simulink model "Pacemaker_final"  (R2020a)
settings: Solver=FixedStepAuto  StartTime=0.0  StopTime=10.0  FixedStep=1e-3  RelTol=1e-3  EnableMultiTasking=on
libraries: etargetslib x17, frdmk64flib x7, simulink x1
(part 1 of 3)
settings Model: ExtModeTrigDuration=5  Creator=Tim_G  LastModifiedBy=Tim_G
settings OptimizationCC: EnhancedBackFolding=on  PassReuseOutputArgsAs=Individual arguments  ZeroExternalMemoryAtStartup=off  ZeroInternalMemoryAtStartup=off  MaxStackSize=64  OptimizeBlockOrder=speed  DifferentSizesBufferReuse=on  OptimizationCustomize=off  EfficientTunableParamExpr=on
settings DebuggingCC: ParameterTunabilityLossMsg=error
settings HardwareCC: ProdBitPerPointer=32  ProdBitPerSizeT=32  ProdBitPerPtrDiffT=32  ProdLargestAtomicInteger=Long  ProdLargestAtomicFloat=Double  ProdEndianess=BigEndian  ProdWordSize=32  ProdHWDeviceType=ARM Compatible->ARM Cortex
settings SFSimCC: MATLABDynamicMemAlloc=off
settings RTWCC: SystemTargetFile=ert.tlc  HardwareBoard=NXP FRDM-K64F  TemplateMakefile=ert_default_tmf  Toolchain=GNU Tools for ARM Embedded Processors
settings CodeAppCC: ForceParamTrailComments=on  IgnoreCustomStorageClasses=off  OperatorAnnotations=on  SimulinkDataObjDesc=on  SFDataObjDesc=on  InsertBlockDesc=on

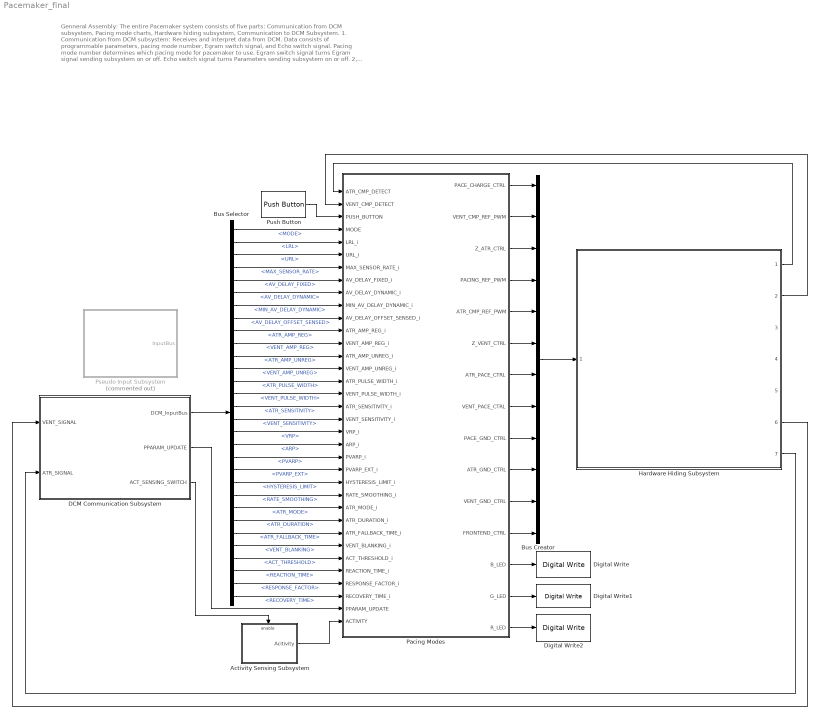
== system Pacemaker_final ==
  note: Genneral Assembly:
      |  The entire Pacemaker system consists of five parts: Communication from DCM subsystem, Pacing mode charts, Hardware hiding subsystem, Communication to DCM Subsystem.
      | 1. Communication from DCM subsystem:
      |       Receives and interpret data from DCM. Data consists of programmable parameters, pacing mode number, Egram switch signal, and Echo switch signal.
      |       Pacing mode number determines which pacing mode for pacemaker to use.
      |       Egram switch signal turns Egram signal sending subsystem on or off.
      |       Echo switch signal turns Parameters sending subsystem on or off.
      | 2, Pacing Modes subsystem:
      |       Implementation of different pacing methods. A multiport switch chooses from which pacing mode to output control signals.
      | 3. Hardware hiding subsystem:
      |       Takes control signals as inputs and sends them to the hardware. Also outputs signals received from the hardware.
      | 4. Communication to DCM Subsystem:
      | 	Sends programmable parameters and/or egram signals to DCM if enable signals (ECHO and/or EGRAM) are turned on.
  Activity Sensing Subsystem : Subsystem
  Bus Creator : BusCreator  Inputs=12
  Bus Selector : BusSelector  OutputSignals=MODE,LRL,URL,MAX_SENSOR_RATE,AV_DELAY_FIXED,AV_DELAY_DYNAMIC,MIN_AV_DELAY_DYNAMIC,AV_DELAY_OFFSET_SENSED,ATR_AMP_REG,VENT_AMP_REG,ATR_AMP_UNREG,VENT_AMP_UNREG,ATR_PULSE_WIDTH,VENT_PULSE_WIDTH,ATR_SENSITIVITY,VENT_SENSITIVITY,VRP,ARP,PVARP,PVARP_EXT,HYSTERESIS_LIMIT,RATE_SMOOTHING,ATR_MODE,ATR_DURATION,ATR_FALLBACK_TIME,VENT_BLANKING,ACT_THRESHOLD,REACTION_TIME,RESPONSE_FACTOR,RECOVERY_TIME
  DCM Communication Subsystem : Subsystem
  Digital Write : frdmk64flib/Digital Write  Whichpin=BLUE_LED
  Digital Write1 : frdmk64flib/Digital Write  Whichpin=GREEN_LED
  Digital Write2 : frdmk64flib/Digital Write  Whichpin=RED_LED
  Hardware Hiding Subsystem : Subsystem  ReferencedSubsystem=k64f_hardware_subsystem
  Pacing Modes : Stateflow chart  TreatAsAtomicUnit=on
      settings: PortSchema="{\"entries\":[{\"content\":{\"sides\":[{\"content\":{\"connectorIds\":[\"In2\",\"In1\",\"In3\",\"In4\",\"In5\",\"In6\",\"In7\",\"In8\",\"In9\",\"In10\",\"In11\",\"In12\",\"In13\",\"In14\",\"In15\",\"In16\",\"In17\",\"In18\",\"In19\",\"In20\",\"In21\",\"In22\",\"In23\",\"In24\",\"In25\",\"In26\",\"In27\",\"In28\",\"In29\",\"In30\",\"In31\",\"In32\",\"In33\",\"In34\",\"In35\"]},\"type\":\"ConnectorPlacement.EquallySpacedRectSide\",\"uuid\":\"6566e723-a8a5-46a2-b90e-16d152fbfa35\"},{\"content\":{\"connectorIds\":[\"Out1\",\"Out2\",\"Out3\",\"Out4\",\"Out5\",\"Out6\",\"Out7\",\"Out8\",\"Out9\",\"Out10\",\"Out11\",\"Out12\",\"Out13\",\"Out14\",\"Out15\"],\"side\":\"RIGHT\"},\"type\":\"ConnectorPlacement.EquallySpacedRectSide\",\"uuid\":\"5fe4a0a7-04e7-4415-b3ec-d211b0e34153\"},{\"content\":{\"connectorIds\":[],\"side\":\"TOP\"},\"type\":\"ConnectorPlacement.EquallySpacedRectSide\",\"uuid\":\"941869fe-4fac-4529-93d8-39aa0ba9c0c9\"}]},\"type\":\"ConnectorPlacement.EquallySpacedConnector\",\"uuid\":\"3c081651-2393-41e1-9361-10a041cf70c8\"}],\"packageUris\":[\"http://schema.mathworks.com/mf0/Connector/19700101\"],\"version\":\"1.0\"}"
  Pseudo Input Subsystem : Subsystem  Commented=on
  Push Button : frdmk64flib/Push Button  Whichswitch=SW2  SampleTime1=-1
  wires:
  Hardware Hiding Subsystem/7 -> DCM Communication Subsystem/2(ATR_SIGNAL)
  Hardware Hiding Subsystem/6 -> DCM Communication Subsystem/1(VENT_SIGNAL)
  Push Button/1 -> Pacing Modes/3(PUSH_BUTTON)
  Hardware Hiding Subsystem/2 -> Pacing Modes/1(VENT_CMP_DETECT)
  Hardware Hiding Subsystem/1 -> Pacing Modes/2(ATR_CMP_DETECT)
  Pacing Modes/1(PACE_CHARGE_CTRL) -> Bus Creator/1
  Pacing Modes/2(VENT_CMP_REF_PWM) -> Bus Creator/2
  Pacing Modes/3(Z_ATR_CTRL) -> Bus Creator/3
  Pacing Modes/4(PACING_REF_PWM) -> Bus Creator/4
  Pacing Modes/5(ATR_CMP_REF_PWM) -> Bus Creator/5
  Pacing Modes/6(Z_VENT_CTRL) -> Bus Creator/6
  Pacing Modes/7(ATR_PACE_CTRL) -> Bus Creator/7
  Pacing Modes/8(VENT_PACE_CTRL) -> Bus Creator/8
  Pacing Modes/9(PACE_GND_CTRL) -> Bus Creator/9
  Pacing Modes/10(ATR_GND_CTRL) -> Bus Creator/10
  Pacing Modes/11(VENT_GND_CTRL) -> Bus Creator/11
  Pacing Modes/12(FRONTEND_CTRL) -> Bus Creator/12
  Bus Creator/1 -> Hardware Hiding Subsystem/1
  DCM Communication Subsystem/1(DCM_InputBus) -> Bus Selector/1
  Bus Selector/1 -> Pacing Modes/4(MODE)  "<MODE>"
  Bus Selector/2 -> Pacing Modes/5(LRL_i)  "<LRL>"
  Bus Selector/3 -> Pacing Modes/6(URL_i)  "<URL>"
  Bus Selector/4 -> Pacing Modes/7(MAX_SENSOR_RATE_i)  "<MAX_SENSOR_RATE>"
  Bus Selector/5 -> Pacing Modes/8(AV_DELAY_FIXED_i)  "<AV_DELAY_FIXED>"
  Bus Selector/6 -> Pacing Modes/9(AV_DELAY_DYNAMIC_i)  "<AV_DELAY_DYNAMIC>"
  Bus Selector/7 -> Pacing Modes/10(MIN_AV_DELAY_DYNAMIC_i)  "<MIN_AV_DELAY_DYNAMIC>"
  Bus Selector/8 -> Pacing Modes/11(AV_DELAY_OFFSET_SENSED_i)  "<AV_DELAY_OFFSET_SENSED>"
  Bus Selector/9 -> Pacing Modes/12(ATR_AMP_REG_i)  "<ATR_AMP_REG>"
  Bus Selector/10 -> Pacing Modes/13(VENT_AMP_REG_i)  "<VENT_AMP_REG>"
  Bus Selector/11 -> Pacing Modes/14(ATR_AMP_UNREG_i)  "<ATR_AMP_UNREG>"
  Bus Selector/12 -> Pacing Modes/15(VENT_AMP_UNREG_i)  "<VENT_AMP_UNREG>"
  Bus Selector/13 -> Pacing Modes/16(ATR_PULSE_WIDTH_i)  "<ATR_PULSE_WIDTH>"
  Bus Selector/14 -> Pacing Modes/17(VENT_PULSE_WIDTH_i)  "<VENT_PULSE_WIDTH>"
  Bus Selector/15 -> Pacing Modes/18(ATR_SENSITIVITY_i)  "<ATR_SENSITIVITY>"
  Bus Selector/16 -> Pacing Modes/19(VENT_SENSITIVITY_i)  "<VENT_SENSITIVITY>"
  Bus Selector/17 -> Pacing Modes/20(VRP_i)  "<VRP>"
  Bus Selector/18 -> Pacing Modes/21(ARP_i)  "<ARP>"
  Bus Selector/19 -> Pacing Modes/22(PVARP_i)  "<PVARP>"
  Bus Selector/20 -> Pacing Modes/23(PVARP_EXT_i)  "<PVARP_EXT>"
  Bus Selector/21 -> Pacing Modes/24(HYSTERESIS_LIMIT_i)  "<HYSTERESIS_LIMIT>"
  Bus Selector/22 -> Pacing Modes/25(RATE_SMOOTHING_i)  "<RATE_SMOOTHING>"
  Bus Selector/23 -> Pacing Modes/26(ATR_MODE_i)  "<ATR_MODE>"
  Bus Selector/24 -> Pacing Modes/27(ATR_DURATION_i)  "<ATR_DURATION>"
  Bus Selector/25 -> Pacing Modes/28(ATR_FALLBACK_TIME_i)  "<ATR_FALLBACK_TIME>"
  Bus Selector/26 -> Pacing Modes/29(VENT_BLANKING_i)  "<VENT_BLANKING>"
  Bus Selector/27 -> Pacing Modes/30(ACT_THRESHOLD_i)  "<ACT_THRESHOLD>"
  Bus Selector/28 -> Pacing Modes/31(REACTION_TIME_i)  "<REACTION_TIME>"
  Bus Selector/29 -> Pacing Modes/32(RESPONSE_FACTOR_i)  "<RESPONSE_FACTOR>"
  Bus Selector/30 -> Pacing Modes/33(RECOVERY_TIME_i)  "<RECOVERY_TIME>"
  Pacing Modes/13(B_LED) -> Digital Write/1
  Pacing Modes/14(G_LED) -> Digital Write1/1
  Pacing Modes/15(R_LED) -> Digital Write2/1
  DCM Communication Subsystem/2(PPARAM_UPDATE) -> Pacing Modes/34(PPARAM_UPDATE)
  Activity Sensing Subsystem/1(Acitivity) -> Pacing Modes/35(ACTIVITY)
  DCM Communication Subsystem/3(ACT_SENSING_SWITCH) -> Activity Sensing Subsystem/Enable

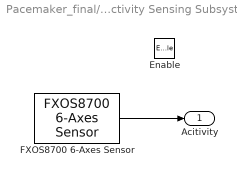
== system Pacemaker_final/Activity Sensing Subsystem ==
  Enable : EnablePort
  FXOS8700 6-Axes Sensor : frdmk64flib/FXOS8700 6-Axes Sensor  Activesensor=Accelerometer only  ODR=800Hz  HybridODR=400Hz  Accelfullrange=-2g to +2g  SampleTime=0.01
  Acitivity : Outport
  wires:
  FXOS8700 6-Axes Sensor/1 -> Acitivity/1

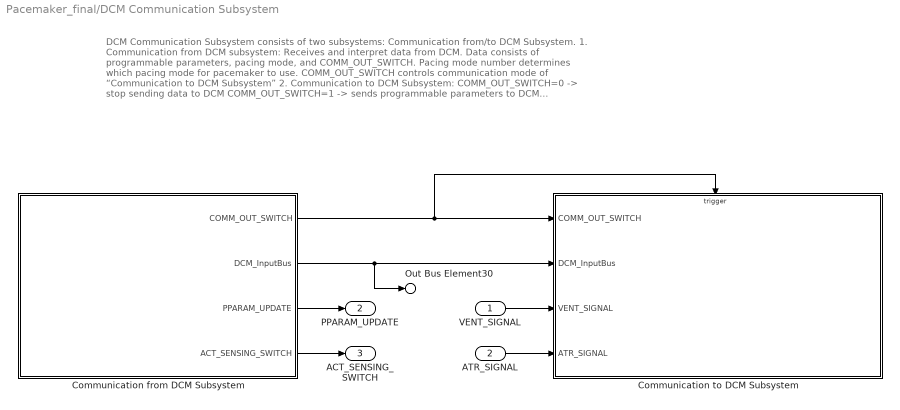
== system Pacemaker_final/DCM Communication Subsystem ==
  note: DCM Communication Subsystem consists of two subsystems: Communication from/to DCM Subsystem.
      | 1. Communication from DCM subsystem:
      | Receives and interpret data from DCM.
      | Data consists of programmable parameters, pacing mode, and COMM_OUT_SWITCH.
      | Pacing mode number determines which pacing mode for pacemaker to use.
      | COMM_OUT_SWITCH controls communication mode of “Communication to DCM Subsystem”
      | 2. Communication to DCM Subsystem:
      | COMM_OUT_SWITCH=0 -> stop sending data to DCM
      | COMM_OUT_SWITCH=1 -> sends programmable parameters to DCM
      | COMM_OUT_SWITCH=2 -> s ends egram signals to DCM
  VENT_SIGNAL : Inport  OutDataTypeStr=double
  ATR_SIGNAL : Inport  Port=2  OutDataTypeStr=double
  Communication from DCM Subsystem : Subsystem
  Communication to DCM Subsystem : Subsystem  TreatAsAtomicUnit=on
  Out Bus Element30 : Outport  PortName=DCM_InputBus
  PPARAM_UPDATE : Outport  Port=2
  ACT_SENSING_SWITCH : Outport  Port=3
  wires:
  VENT_SIGNAL/1 -> Communication to DCM Subsystem/3(VENT_SIGNAL)
  ATR_SIGNAL/1 -> Communication to DCM Subsystem/4(ATR_SIGNAL)
  Communication from DCM Subsystem/3(PPARAM_UPDATE) -> PPARAM_UPDATE/1
  Communication from DCM Subsystem/1(COMM_OUT_SWITCH) -> Communication to DCM Subsystem/Trigger, Communication to DCM Subsystem/1(COMM_OUT_SWITCH)
  Communication from DCM Subsystem/4(ACT_SENSING_SWITCH) -> ACT_SENSING_SWITCH/1
  Communication from DCM Subsystem/2(DCM_InputBus) -> Out Bus Element30/1, Communication to DCM Subsystem/2(DCM_InputBus)

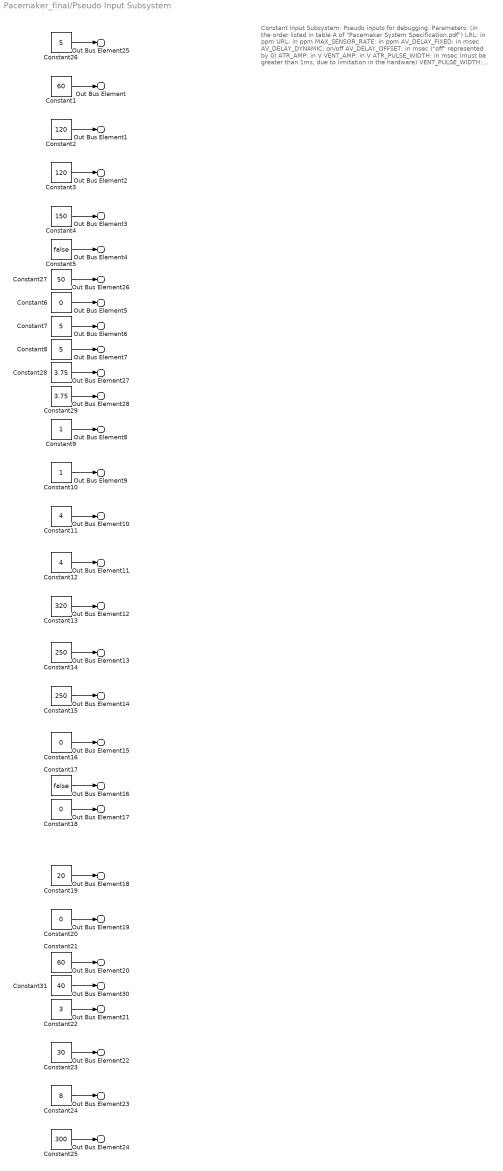
== system Pacemaker_final/Pseudo Input Subsystem ==
  note: Constant Input Subsystem:
      | Pseudo inputs for debugging.
      |
      | Parameters:
      | (in the order listed in table A of "Pacemaker System Specification.pdf")
      | LRL: in ppm
      | URL: in ppm
      | MAX_SENSOR_RATE: in ppm
      | AV_DELAY_FIXED: in msec
      | AV_DELAY_DYNAMIC: on/off
      | AV_DELAY_OFFSET: in msec ("off" represented by 0)
      | ATR_AMP: in V
      | VENT_AMP: in V
      | ATR_PULSE_WIDTH: in msec (must be greater than 1ms, due to
      | limitation in the hardware)
      | VENT_PULSE_WIDTH: in msec
      | ATR_SENSITIVITY: in V
      | VENT_SENSITIVITY: in V
      | VRP: in msec
      | ARP: in msec
      | PVARP: in msec
      | PVARP_EXT: in msec ("off" represented by 0)
      | HYSTERESIS: off/same choices as LRL (represented by "on")
      | RATE_SMOOTHING: off represented by 0
      | ATR_DURATION: in cardiac cycles
      | ATR_FALLBACK_MODE
      | ATR_FALLBACK_TIME: in sec
      | ACT_THRESHOLD:
      | 0-V-Low
      | 1-Low
      | 2-Med-Low
      | 3-Med
      | 4-Med-High
      | 5-High
      | 6-V-High
      | REACTION_TIME: in sec
      | RESPONSE_FACTOR
      | RECOVERY_TIME: in sec
  Constant1 : Constant  Value=60
  Constant10 : Constant
  Constant11 : Constant  Value=4
  Constant12 : Constant  Value=4
  Constant13 : Constant  Value=320
  Constant14 : Constant  Value=250
  Constant15 : Constant  Value=250
  Constant{6,16,18,20} (4 alike) : Constant  Value=0
  Constant17 : Constant  Value=false
  Constant19 : Constant  Value=20
  Constant2 : Constant  Value=120
  Constant21 : Constant  Value=60
  Constant22 : Constant  Value=3
  Constant23 : Constant  Value=30
  Constant24 : Constant  Value=8
  Constant25 : Constant  Value=300
  Constant26 : Constant  Value=5
  Constant27 : Constant  Value=50
  Constant28 : Constant  Value=3.75
  Constant29 : Constant  Value=3.75
  Constant3 : Constant  Value=120
  Constant31 : Constant  Value=40
  Constant4 : Constant  Value=150
  Constant5 : Constant  Value=false
  Constant7 : Constant  Value=5
  Constant8 : Constant  Value=5
  Constant9 : Constant
  Out Bus Element : Outport  PortName=InputBus  Element=LRL
  Out Bus Element1 : Outport  PortName=InputBus  Element=URL
  Out Bus Element2 : Outport  PortName=InputBus  Element=MAX_SENSOR_RATE
  Out Bus Element3 : Outport  PortName=InputBus  Element=AV_DELAY_FIXED
  Out Bus Element4 : Outport  PortName=InputBus  Element=AV_DELAY_DYNAMIC
  Out Bus Element5 : Outport  PortName=InputBus  Element=AV_DELAY_OFFSET_SENSED
  Out Bus Element6 : Outport  PortName=InputBus  Element=ATR_AMP_REG
  Out Bus Element7 : Outport  PortName=InputBus  Element=VENT_AMP_REG
  Out Bus Element8 : Outport  PortName=InputBus  Element=ATR_PULSE_WIDTH
  Out Bus Element9 : Outport  PortName=InputBus  Element=VENT_PULSE_WIDTH
  Out Bus Element10 : Outport  PortName=InputBus  Element=ATR_SENSITIVITY
  Out Bus Element11 : Outport  PortName=InputBus  Element=VENT_SENSITIVITY
  Out Bus Element12 : Outport  PortName=InputBus  Element=VRP
  Out Bus Element13 : Outport  PortName=InputBus  Element=ARP
  Out Bus Element14 : Outport  PortName=InputBus  Element=PVARP
  Out Bus Element15 : Outport  PortName=InputBus  Element=PVARP_EXT
  Out Bus Element16 : Outport  PortName=InputBus  Element=HYSTERESIS
  Out Bus Element17 : Outport  PortName=InputBus  Element=RATE_SMOOTHING
  Out Bus Element18 : Outport  PortName=InputBus  Element=ATR_DURATION
  Out Bus Element19 : Outport  PortName=InputBus  Element=ATR_FALLBACK_MODE
  Out Bus Element20 : Outport  PortName=InputBus  Element=ATR_FALLBACK_TIME
  Out Bus Element21 : Outport  PortName=InputBus  Element=ACT_THRESHOLD
  Out Bus Element22 : Outport  PortName=InputBus  Element=REACTION_TIME
  Out Bus Element23 : Outport  PortName=InputBus  Element=RESPONSE_FACTOR
  Out Bus Element24 : Outport  PortName=InputBus  Element=RECOVERY_TIME
  Out Bus Element25 : Outport  PortName=InputBus  Element=MODE
  Out Bus Element26 : Outport  PortName=InputBus  Element=MIN_AV_DELAY_DYNAMIC
  Out Bus Element27 : Outport  PortName=InputBus  Element=ATR_AMP_UNREG
  Out Bus Element28 : Outport  PortName=InputBus  Element=VENT_AMP_UNREG
  Out Bus Element30 : Outport  PortName=InputBus  Element=VENT_BLANKING
  wires:
  Constant1/1 -> Out Bus Element/1
  Constant2/1 -> Out Bus Element1/1
  Constant4/1 -> Out Bus Element3/1
  Constant3/1 -> Out Bus Element2/1
  Constant5/1 -> Out Bus Element4/1
  Constant6/1 -> Out Bus Element5/1
  Constant8/1 -> Out Bus Element7/1
  Constant7/1 -> Out Bus Element6/1
  Constant10/1 -> Out Bus Element9/1
  Constant11/1 -> Out Bus Element10/1
  Constant9/1 -> Out Bus Element8/1
  Constant13/1 -> Out Bus Element12/1
  Constant12/1 -> Out Bus Element11/1
  Constant14/1 -> Out Bus Element13/1
  Constant15/1 -> Out Bus Element14/1
  Constant19/1 -> Out Bus Element18/1
  Constant18/1 -> Out Bus Element17/1
  Constant16/1 -> Out Bus Element15/1
  Constant17/1 -> Out Bus Element16/1
  Constant25/1 -> Out Bus Element24/1
  Constant24/1 -> Out Bus Element23/1
  Constant23/1 -> Out Bus Element22/1
  Constant22/1 -> Out Bus Element21/1
  Constant20/1 -> Out Bus Element19/1
  Constant21/1 -> Out Bus Element20/1
  Constant26/1 -> Out Bus Element25/1
  Constant27/1 -> Out Bus Element26/1
  Constant28/1 -> Out Bus Element27/1
  Constant29/1 -> Out Bus Element28/1
  Constant31/1 -> Out Bus Element30/1

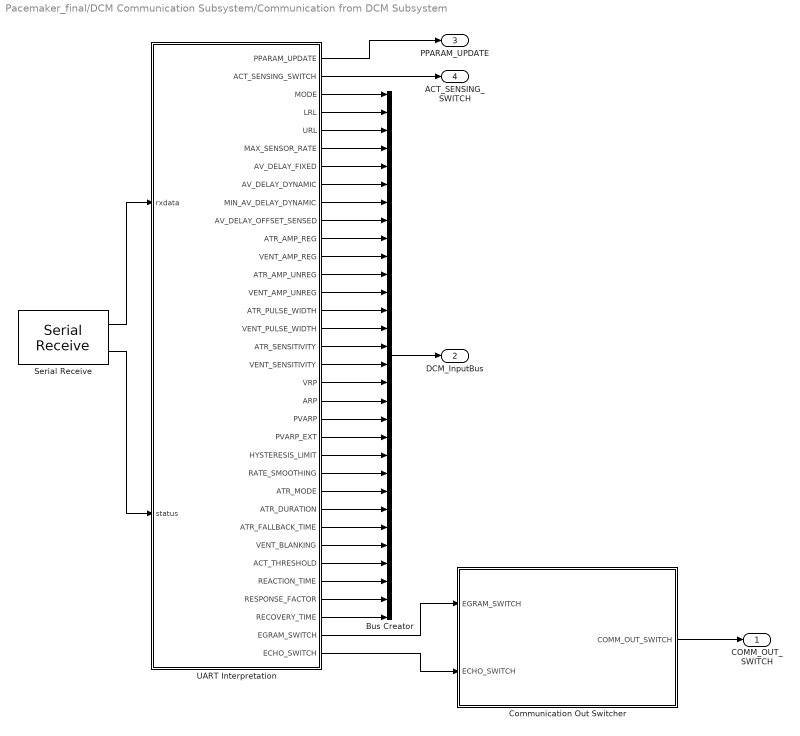
== system Pacemaker_final/DCM Communication Subsystem/Communication from DCM Subsystem ==
  Bus Creator : BusCreator  Inputs=30
  Communication Out Switcher : Stateflow chart  TreatAsAtomicUnit=on
  Serial Receive : frdmk64flib/Serial Receive  SCIModule=0  Baudrate=uint32(9600)  Parity=None  StopBits=1  HardwareFlowControl=None  ByteOrder=LittleEndian  DataType=uint8  DataLength=59  BlockingMode=off  OutputStatus=on  SampleTime=-1
  UART Interpretation : Stateflow chart  TreatAsAtomicUnit=on
      settings: PortSchema="{\"entries\":[{\"content\":{\"sides\":[{\"content\":{\"connectorIds\":[\"In1\",\"In2\"]},\"type\":\"ConnectorPlacement.EquallySpacedRectSide\",\"uuid\":\"8bf45b7e-957d-4d49-8afa-52d597e5211b\"},{\"content\":{\"connectorIds\":[\"Out33\",\"Out34\",\"Out1\",\"Out2\",\"Out3\",\"Out4\",\"Out5\",\"Out6\",\"Out7\",\"Out8\",\"Out9\",\"Out10\",\"Out11\",\"Out12\",\"Out13\",\"Out14\",\"Out15\",\"Out16\",\"Out17\",\"Out18\",\"Out19\",\"Out20\",\"Out21\",\"Out22\",\"Out23\",\"Out24\",\"Out25\",\"Out26\",\"Out27\",\"Out28\",\"Out29\",\"Out30\",\"Out31\",\"Out32\"],\"side\":\"RIGHT\"},\"type\":\"ConnectorPlacement.EquallySpacedRectSide\",\"uuid\":\"d38d0b56-01b9-48e9-aa1c-1551120d845a\"},{\"content\":{\"connectorIds\":[],\"side\":\"TOP\"},\"type\":\"ConnectorPlacement.EquallySpacedRectSide\",\"uuid\":\"18196cd6-21fd-4409-aed1-274194e36cea\"}]},\"type\":\"ConnectorPlacement.EquallySpacedConnector\",\"uuid\":\"d120a801-f3dc-4c99-bead-ec7f8e612754\"}],\"packageUris\":[\"http://schema.mathworks.com/mf0/Connector/19700101\"],\"version\":\"1.0\"}"
  COMM_OUT_SWITCH : Outport
  DCM_InputBus : Outport  Port=2
  PPARAM_UPDATE : Outport  Port=3
  ACT_SENSING_SWITCH : Outport  Port=4
  wires:
  UART Interpretation/5(AV_DELAY_FIXED) -> Bus Creator/5
  UART Interpretation/14(VENT_PULSE_WIDTH) -> Bus Creator/14
  UART Interpretation/10(VENT_AMP_REG) -> Bus Creator/10
  UART Interpretation/17(VRP) -> Bus Creator/17
  UART Interpretation/6(AV_DELAY_DYNAMIC) -> Bus Creator/6
  UART Interpretation/9(ATR_AMP_REG) -> Bus Creator/9
  UART Interpretation/27(ACT_THRESHOLD) -> Bus Creator/27
  UART Interpretation/24(ATR_DURATION) -> Bus Creator/24
  UART Interpretation/18(ARP) -> Bus Creator/18
  UART Interpretation/8(AV_DELAY_OFFSET_SENSED) -> Bus Creator/8
  UART Interpretation/7(MIN_AV_DELAY_DYNAMIC) -> Bus Creator/7
  Serial Receive/2 -> UART Interpretation/2(status)
  UART Interpretation/3(URL) -> Bus Creator/3
  UART Interpretation/26(VENT_BLANKING) -> Bus Creator/26
  UART Interpretation/13(ATR_PULSE_WIDTH) -> Bus Creator/13
  UART Interpretation/15(ATR_SENSITIVITY) -> Bus Creator/15
  UART Interpretation/11(ATR_AMP_UNREG) -> Bus Creator/11
  UART Interpretation/16(VENT_SENSITIVITY) -> Bus Creator/16
  UART Interpretation/30(RECOVERY_TIME) -> Bus Creator/30
  UART Interpretation/20(PVARP_EXT) -> Bus Creator/20
  UART Interpretation/29(RESPONSE_FACTOR) -> Bus Creator/29
  UART Interpretation/19(PVARP) -> Bus Creator/19
  Serial Receive/1 -> UART Interpretation/1(rxdata)
  UART Interpretation/4(MAX_SENSOR_RATE) -> Bus Creator/4
  UART Interpretation/23(ATR_MODE) -> Bus Creator/23
  UART Interpretation/22(RATE_SMOOTHING) -> Bus Creator/22
  UART Interpretation/12(VENT_AMP_UNREG) -> Bus Creator/12
  UART Interpretation/28(REACTION_TIME) -> Bus Creator/28
  UART Interpretation/25(ATR_FALLBACK_TIME) -> Bus Creator/25
  UART Interpretation/21(HYSTERESIS_LIMIT) -> Bus Creator/21
  UART Interpretation/2(LRL) -> Bus Creator/2
  UART Interpretation/1(MODE) -> Bus Creator/1
  Bus Creator/1 -> DCM_InputBus/1
  Communication Out Switcher/1(COMM_OUT_SWITCH) -> COMM_OUT_SWITCH/1
  UART Interpretation/31(EGRAM_SWITCH) -> Communication Out Switcher/1(EGRAM_SWITCH)
  UART Interpretation/32(ECHO_SWITCH) -> Communication Out Switcher/2(ECHO_SWITCH)
  UART Interpretation/33(PPARAM_UPDATE) -> PPARAM_UPDATE/1
  UART Interpretation/34(ACT_SENSING_SWITCH) -> ACT_SENSING_SWITCH/1

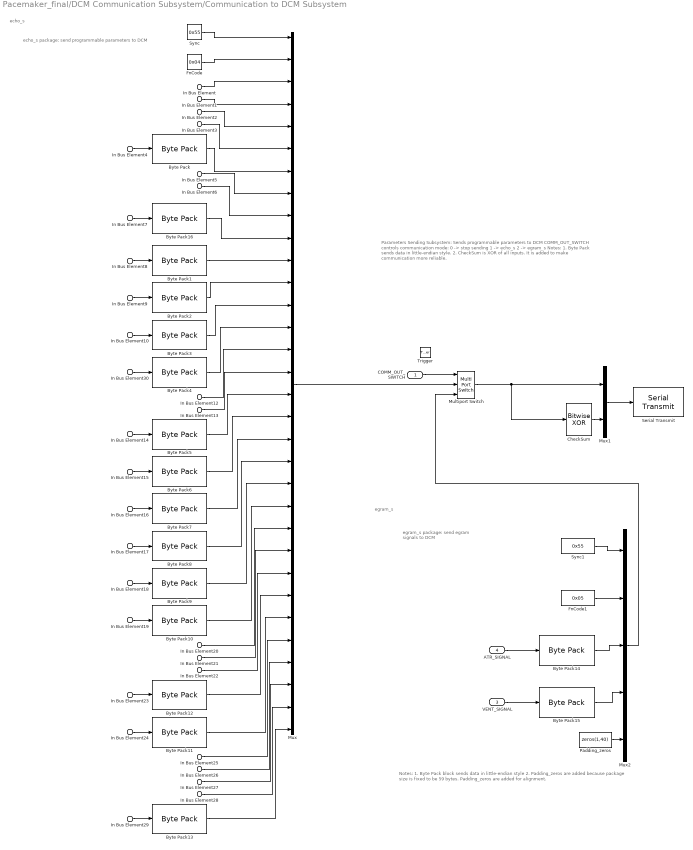
== system Pacemaker_final/DCM Communication Subsystem/Communication to DCM Subsystem ==
  note: egram_s package:
      | send egram signals to DCM
  note: echo_s package:
      | send programmable parameters to DCM
  note: echo_s
  note: egram_s
  note: Parameters Sending Subsystem:
      | Sends programmable parameters to DCM
      | COMM_OUT_SWITCH controls communication mode:
      | 0 -> stop sending
      | 1 -> echo_s
      | 2 -> egram_s
      | Notes:
      | 1. Byte Pack sends data in little-endian style.
      | 2. CheckSum is XOR of all inputs. It is added to make communication more reliable.
  note: Notes:
      | 1. Byte Pack block sends data in little-endian style
      | 2. Padding_zeros are added because package size is fixed to be 59 bytes. Padding_zeros are added for alignment.
  COMM_OUT_SWITCH : Inport
  In Bus Element : Inport  Port=2  PortName=DCM_InputBus  Element=MODE
  In Bus Element1 : Inport  Port=2  PortName=DCM_InputBus  Element=LRL
  In Bus Element2 : Inport  Port=2  PortName=DCM_InputBus  Element=URL
  In Bus Element3 : Inport  Port=2  PortName=DCM_InputBus  Element=MAX_SENSOR_RATE
  In Bus Element4 : Inport  Port=2  PortName=DCM_InputBus  Element=AV_DELAY_FIXED
  In Bus Element5 : Inport  Port=2  PortName=DCM_InputBus  Element=AV_DELAY_DYNAMIC
  In Bus Element6 : Inport  Port=2  PortName=DCM_InputBus  Element=MIN_AV_DELAY_DYNAMIC
  In Bus Element7 : Inport  Port=2  PortName=DCM_InputBus  Element=AV_DELAY_OFFSET_SENSED
  In Bus Element8 : Inport  Port=2  PortName=DCM_InputBus  Element=ATR_AMP_REG
  In Bus Element9 : Inport  Port=2  PortName=DCM_InputBus  Element=VENT_AMP_REG
  In Bus Element10 : Inport  Port=2  PortName=DCM_InputBus  Element=ATR_AMP_UNREG
  In Bus Element12 : Inport  Port=2  PortName=DCM_InputBus  Element=ATR_PULSE_WIDTH
  In Bus Element13 : Inport  Port=2  PortName=DCM_InputBus  Element=VENT_PULSE_WIDTH
  In Bus Element14 : Inport  Port=2  PortName=DCM_InputBus  Element=ATR_SENSITIVITY
  In Bus Element15 : Inport  Port=2  PortName=DCM_InputBus  Element=VENT_SENSITIVITY
  In Bus Element16 : Inport  Port=2  PortName=DCM_InputBus  Element=VRP
  In Bus Element17 : Inport  Port=2  PortName=DCM_InputBus  Element=ARP
  In Bus Element18 : Inport  Port=2  PortName=DCM_InputBus  Element=PVARP
  In Bus Element19 : Inport  Port=2  PortName=DCM_InputBus  Element=PVARP_EXT
  In Bus Element20 : Inport  Port=2  PortName=DCM_InputBus  Element=HYSTERESIS_LIMIT
  In Bus Element21 : Inport  Port=2  PortName=DCM_InputBus  Element=RATE_SMOOTHING
  In Bus Element22 : Inport  Port=2  PortName=DCM_InputBus  Element=ATR_MODE
  In Bus Element23 : Inport  Port=2  PortName=DCM_InputBus  Element=ATR_DURATION
  In Bus Element24 : Inport  Port=2  PortName=DCM_InputBus  Element=ATR_FALLBACK_TIME
  In Bus Element25 : Inport  Port=2  PortName=DCM_InputBus  Element=VENT_BLANKING
  In Bus Element26 : Inport  Port=2  PortName=DCM_InputBus  Element=ACT_THRESHOLD
  In Bus Element27 : Inport  Port=2  PortName=DCM_InputBus  Element=REACTION_TIME
  In Bus Element28 : Inport  Port=2  PortName=DCM_InputBus  Element=RESPONSE_FACTOR
  In Bus Element29 : Inport  Port=2  PortName=DCM_InputBus  Element=RECOVERY_TIME
  In Bus Element30 : Inport  Port=2  PortName=DCM_InputBus  Element=VENT_AMP_UNREG
  VENT_SIGNAL : Inport  Port=3  OutDataTypeStr=double
  ATR_SIGNAL : Inport  Port=4  OutDataTypeStr=double
  Trigger : TriggerPort  VariantControl=Variant  InitialTriggerSignalState=zero  PortDimensions=1
  Byte Pack{,7..13} (8 alike) : etargetslib/Byte Pack  datatypes={'uint16'}  byteAlign=1
  Byte Pack{1..6} (6 alike) : etargetslib/Byte Pack  datatypes={'single'}  byteAlign=1
  Byte Pack14 : etargetslib/Byte Pack  datatypes={'double'}  byteAlign=1
  Byte Pack15 : etargetslib/Byte Pack  datatypes={'double'}  byteAlign=1
  Byte Pack16 : etargetslib/Byte Pack  datatypes={'int8'}  byteAlign=1
  CheckSum : simulink/Logic and Bit Operations/Bitwise Operator  logicop=XOR  UseBitMask=off  BitMask=bin2dec('11011001')  BitMaskRealWorld=Stored Integer
  FnCode : Constant  Value=0x04  OutDataTypeStr=uint8
  FnCode1 : Constant  Value=0x05  OutDataTypeStr=uint8
  Multiport Switch : MultiPortSwitch  Inputs=2
  Mux : Mux  Inputs=32
  Mux1 : Mux  Inputs=2
  Mux2 : Mux  Inputs=5
  Padding_zeros : Constant  Value=zeros(1,40)  VectorParams1D=off  OutDataTypeStr=uint8
  Serial Transmit : frdmk64flib/Serial Transmit  SCIModule=0  Baudrate=uint32(9600)  Parity=None  StopBits=1  HardwareFlowControl=None  ByteOrder=LittleEndian  BlockingMode=on  OutputStatus=off
  Sync : Constant  Value=0x55  OutDataTypeStr=uint8
  Sync1 : Constant  Value=0x55  OutDataTypeStr=uint8
  wires:
  In Bus Element25/1 -> Mux/28
  Byte Pack13/1 -> Mux/32
  Byte Pack11/1 -> Mux/27
  In Bus Element20/1 -> Mux/23
  Byte Pack12/1 -> Mux/26
  Byte Pack8/1 -> Mux/20
  Byte Pack10/1 -> Mux/22
  In Bus Element/1 -> Mux/3
  Byte Pack9/1 -> Mux/21
  Byte Pack7/1 -> Mux/19
  Byte Pack5/1 -> Mux/17
  In Bus Element12/1 -> Mux/15
  Byte Pack1/1 -> Mux/11
  Byte Pack6/1 -> Mux/18
  In Bus Element6/1 -> Mux/9
  In Bus Element26/1 -> Mux/29
  Byte Pack3/1 -> Mux/13
  Byte Pack2/1 -> Mux/12
  Byte Pack/1 -> Mux/7
  In Bus Element21/1 -> Mux/24
  In Bus Element22/1 -> Mux/25
  In Bus Element28/1 -> Mux/31
  In Bus Element27/1 -> Mux/30
  Byte Pack4/1 -> Mux/14
  In Bus Element13/1 -> Mux/16
  In Bus Element5/1 -> Mux/8
  In Bus Element1/1 -> Mux/4
  In Bus Element4/1 -> Byte Pack/1
  In Bus Element3/1 -> Mux/6
  In Bus Element2/1 -> Mux/5
  FnCode/1 -> Mux/2
  Sync/1 -> Mux/1
  Mux1/1 -> Serial Transmit/1
  CheckSum/1 -> Mux1/2
  Sync1/1 -> Mux2/1
  Mux/1 -> Multiport Switch/2
  Multiport Switch/1 -> CheckSum/1, Mux1/1
  Byte Pack14/1 -> Mux2/3
  Byte Pack15/1 -> Mux2/4
  FnCode1/1 -> Mux2/2
  Mux2/1 -> Multiport Switch/3
  Padding_zeros/1 -> Mux2/5
  Byte Pack16/1 -> Mux/10
  In Bus Element7/1 -> Byte Pack16/1
  In Bus Element8/1 -> Byte Pack1/1
  In Bus Element9/1 -> Byte Pack2/1
  In Bus Element10/1 -> Byte Pack3/1
  In Bus Element30/1 -> Byte Pack4/1
  In Bus Element14/1 -> Byte Pack5/1
  In Bus Element15/1 -> Byte Pack6/1
  In Bus Element16/1 -> Byte Pack7/1
  In Bus Element17/1 -> Byte Pack8/1
  In Bus Element18/1 -> Byte Pack9/1
  In Bus Element19/1 -> Byte Pack10/1
  In Bus Element29/1 -> Byte Pack13/1
  In Bus Element23/1 -> Byte Pack12/1
  In Bus Element24/1 -> Byte Pack11/1
  ATR_SIGNAL/1 -> Byte Pack14/1
  VENT_SIGNAL/1 -> Byte Pack15/1
  COMM_OUT_SWITCH/1 -> Multiport Switch/1
